simulink model "PID_control_blockl"  (R2020b)
settings: Solver=ode45  StartTime=0.0  StopTime=120  RelTol=1e-3
values from neighbouring files (symbols this model uses):
  b = 50    [parameters.m]
  Ki = 40    [parameters.m]
  Kp = 800    [parameters.m]
  m = 1000    [parameters.m]
settings Model: Creator=baner  LastModifiedBy=baner

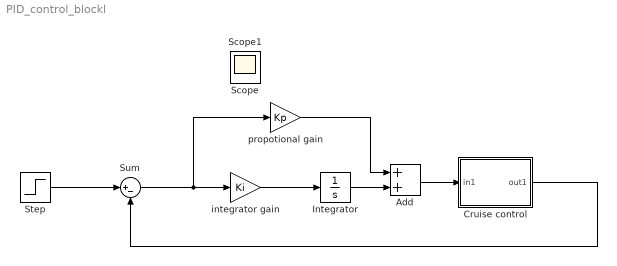
== system PID_control_blockl ==
  Add : Sum
  "Cruise control " : Subsystem
  Integrator : Integrator
  Step : Step  SampleTime=0
  Sum : Sum  Inputs=|+-
  integrator gain : Gain  Gain=Ki
  propotional gain : Gain  Gain=Kp
  Scope : Scope
  Scope1 : Scope
  wires:
  Sum/1 -> integrator gain/1, propotional gain/1
  integrator gain/1 -> Integrator/1
  "Cruise control "/1(out1) -> Sum/2
  Integrator/1 -> Add/2
  propotional gain/1 -> Add/1
  Add/1 -> "Cruise control "/1(in1)
  Step/1 -> Sum/1

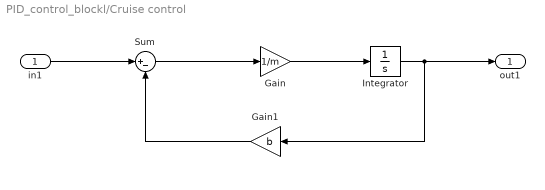
== system PID_control_blockl/Cruise control  ==
  in1 : Inport
  Gain : Gain  Gain=1/m
  Gain1 : Gain  Gain=b
  Integrator : Integrator
  Sum : Sum  Inputs=|+-
  out1 : Outport
  wires:
  Gain1/1 -> Sum/2
  Integrator/1 -> out1/1, Gain1/1
  Sum/1 -> Gain/1
  Gain/1 -> Integrator/1
  in1/1 -> Sum/1
